simulink model "BR_GATES_HDL"  (R2016a)
settings: Solver=FixedStepDiscrete  SolverMode=SingleTasking  StartTime=0.0  StopTime=20  FixedStep=1  RelTol=1e-3
libraries: simulink x1
settings Model: Creator=YankinYY  LastModifiedBy=YankinYY
settings DataIOCC: LimitDataPoints=on  SaveFormat=Array
settings OptimizationCC: BlockReduction=off  ConditionallyExecuteInputs=off  DefaultParameterBehavior=Inlined
settings DebuggingCC: AlgebraicLoopMsg=error  SolverPrmCheckMsg=warning
settings HardwareCC: ProdBitPerPointer=32  ProdLargestAtomicFloat=None  ProdIntDivRoundTo=Undefined  ProdEndianess=Unspecified  ProdWordSize=32  ProdHWDeviceType=ASIC/FPGA->ASIC/FPGA  ProdEqTarget=off
settings ModelReferenceCC: PropagateSignalLabelsOutOfModel=off
settings ConfigComp: CovEnable=on  CovScope=Subsystem  RecordCoverage=on  CovPath=BR_GATES_CH  CovMetricSettings=dcmw  CovHTMLOptions=-sRT=1 -sVT=0 -aTS=1 -bRG=1 -bTC=1 -hTR=0 -nFC=0 -nFD=1 -scm=1 -bcm=1 -xEv=0 -xEM=0  CovModelRefEnable=Off  CovSFcnEnable=off

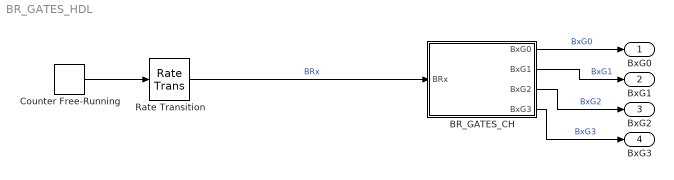
== system BR_GATES_HDL ==
  BR_GATES_CH : Stateflow chart  TreatAsAtomicUnit=on
  Counter Free-Running : simulink/Sources/Counter Free-Running  NumBits=4  tsamp=4
  Rate Transition : RateTransition  Deterministic=off
  BxG0 : Outport
  BxG1 : Outport  Port=2
  BxG2 : Outport  Port=3
  BxG3 : Outport  Port=4
  wires:
  Rate Transition/1 -> BR_GATES_CH/1(BRx)  "BRx"
  BR_GATES_CH/4(BxG3) -> BxG3/1  "BxG3"
  BR_GATES_CH/3(BxG2) -> BxG2/1  "BxG2"
  BR_GATES_CH/2(BxG1) -> BxG1/1  "BxG1"
  BR_GATES_CH/1(BxG0) -> BxG0/1  "BxG0"
  Counter Free-Running/1 -> Rate Transition/1

== stateflow chart BR_GATES_HDL/BR_GATES_CH ==
  settings: updateMethod=DISCRETE  sampleTime=1  executeAtInitialization=1
  state G0_G1 [parallel]
    settings: executionOrder=1
    state B1
      state OFF
        en: BxG0 = 0;...
        BxG1 = 1;
      state dt
        en: BxG1 = 0;
      state dt1
        en: BxG0 = 0;
      state ON
        en: BxG0 = 1;...
        BxG1 = 0;
      G0_G1.B1.OFF -> G0_G1.B1.dt : [BRx == 1 || ...
          | BRx == 4]
      G0_G1.B1.dt1 -> G0_G1.B1.OFF : [after(dt,tick)]
      G0_G1.B1.dt -> G0_G1.B1.ON : [after(dt,tick)]
      G0_G1.B1.ON -> G0_G1.B1.dt1 : [BRx == 2 || ...
          | BRx == 3]
    state tri_state
      en: BxG0 = 0;...
      BxG1 = 0;
    G0_G1.tri_state -> G0_G1.B1.OFF [order 2] : [BRx == 2 || ...
        | BRx == 3]
    (default) -> G0_G1.tri_state
    G0_G1.B1 -> G0_G1.tri_state : [BRx == 0]
    G0_G1.tri_state -> G0_G1.B1.ON [order 1] : [BRx == 1 || ...
        | BRx == 4]
  state G2_G3 [parallel]
    settings: executionOrder=2
    state B1
      state OFF
        en: BxG2 = 0;...
        BxG3 = 1;
      state dt
        BxG3 = 0;
      state dt1
        en: BxG2 = 0;
      state ON
        en: BxG2 = 1;...
        BxG3 = 0;
      G2_G3.B1.OFF -> G2_G3.B1.dt : [BRx == 3 || ...
          | BRx == 4]
      G2_G3.B1.dt1 -> G2_G3.B1.OFF : [after(dt,tick)]
      G2_G3.B1.dt -> G2_G3.B1.ON : [after(dt,tick)]
      G2_G3.B1.ON -> G2_G3.B1.dt1 : [BRx == 1 || ...
          | BRx == 2]
    state tri_state
      en: BxG2 = 0;...
      BxG3 = 0;
    G2_G3.tri_state -> G2_G3.B1.OFF [order 2] : [BRx == 1 || ...
        | BRx == 2]
    (default) -> G2_G3.tri_state
    G2_G3.B1 -> G2_G3.tri_state : [BRx == 0]
    G2_G3.tri_state -> G2_G3.B1.ON [order 1] : [BRx == 3 || ...
        | BRx == 4]
  data: BRx input fixdt(0,4,0); BxG0 output fixdt(0,1,0); BxG1 output fixdt(0,1,0); BxG2 output fixdt(0,1,0); BxG3 output fixdt(0,1,0); dt constant uint8 =1
  data BRx settings: description=|
      | 0000b - все транзисторы разомкнуты 0
      | 0001b - замкнуты транизсторы левой диагонали (G0, G3) 1
      | 0010b - замкнуты оба нижних транзистора (G1, G3) 2
      | 0011b - замкнуты транзисторы правой диагонали (G2, G1) 3
      | 0100b - замкнуты оба верхних транзистора (G0, G2) 4
  data BxG0 settings: description=открытому состоянию ключа соответствует низкий логический уровень (инвертор в Quartus)
  data BxG2 settings: description=открытому состоянию ключа соответствует низкий логический уровень (инвертор в Quartus)
  data dt settings: description=dead-time в отсчетах
